simulink model "CDPRSim"  (R2023a)
settings: Solver=FixedStepAuto  StartTime=0.0  StopTime=inf  FixedStep=0.0001  RelTol=1e-3
values from neighbouring files (symbols this model uses):
  x11 = input('Enter x11 ')    [CDPRm.m]
  y11 = input('Enter y11 ')    [CDPRm.m]
undefined symbols (not defined in the file or in its folder): LBA, LTA, RBA, RTA
libraries: dspmathops x2, vrlib x1
(part 1 of 2)
settings Model: Creator=user  LastModifiedBy=omert
settings SolverCC: AlgebraicLoopSolver=TrustRegion
settings DataIOCC: ReturnWorkspaceOutputs=off
settings DebuggingCC: UnconnectedInputMsg=warning  UnconnectedOutputMsg=warning  UnconnectedLineMsg=warning  ArithmeticOperatorsInVariantConditions=warning
settings ModelReferenceCC: EnableRefExpFcnMdlSchedulingChecks=on
settings SFSimCC: CustomCodeUndefinedFunction=UseInterfaceOnly

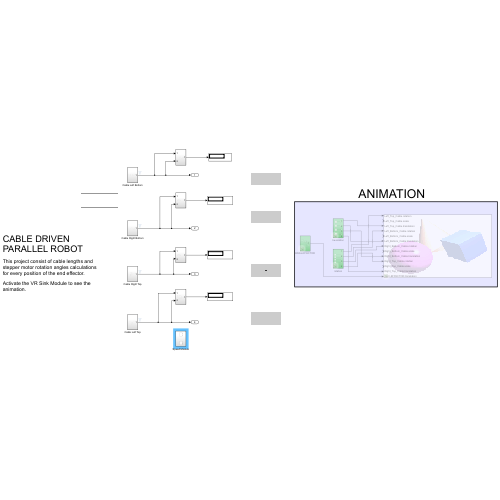
[thumbnail: Simulink's stored preview of the top-level diagram]
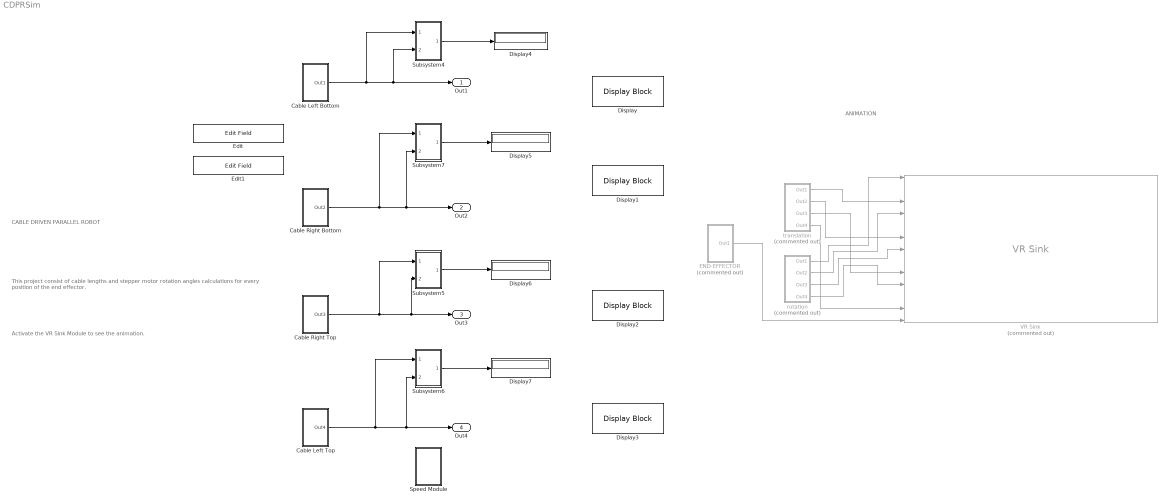
== system CDPRSim ==
  note: ANIMATION
  note: This project consist of cable lengths and stepper motor rotation angles calculations
      | for every position of the end effector.
  note: CABLE DRIVEN PARALLEL ROBOT
  note: Activate the VR Sink Module to see the
      | animation.
  Cable Left Bottom : Subsystem
  Cable Left Top : Subsystem
  Cable Right Bottom : Subsystem
  Cable Right Top : Subsystem
  Display{,1..3} (4 alike) : DisplayBlock  LabelPosition=Hide  Format=long
  Display{4..7} (4 alike) : Display
  END-EFFECTOR : Subsystem  Commented=on
  Edit : EditField  LabelPosition=Hide  ShowInitialText=on  Alignment=Center
  Edit1 : EditField  LabelPosition=Hide  ShowInitialText=on  Alignment=Center
  Speed Module : Subsystem
  Subsystem4 : Subsystem
  Subsystem5 : Subsystem
  Subsystem6 : Subsystem
  Subsystem7 : Subsystem
  VR Sink : vrlib/VR Sink  Commented=on  InstantiateOnLoad=on  SampleTime=0.00000000000000000000001  ViewEnable=on  RemoteChange=off  RemoteView=off  FieldsWritten=Left_Top_Cable.rotation.4.1.1.double#Left_Top_Cable.scale.3.1.1.double#Left_Top_Cable.translation.3.1.1.double#Left_Bottom_Cable.rotation.4.1.1.double#Left_Bottom_Cable.scale.3.1.1.double#Left_Bottom_Cable.translation.3.1.1.double#Right_Bottom_Cable.rotation.4.1.1.double#Right_Bottom_Cable.scale.3.1.1.double#Right_Bottom_Cable.translation.3.1.1.double#Right_Top_Cable.rotation.4.1.1.double#Right_Top_Cable.scale.3.1.1.double#Right_Top_Cable.translation.3.1.1.double#END-EFFECTOR.translation.3.1.1.double  WorldFileName=C:\Users\omert\OneDrive\Masaüstü\EFSANE.WRL  AutoView=off  VideoDimensions=[]  AllowVariableSize=off  FigureProperties="{'Position', 'Name', 'Viewpoint', 'CameraBound', 'CameraDirection', 'CameraPosition', 'CameraUpVector', 'ZoomFactor', 'Antialiasing', 'Headlight', 'Lighting', 'NavPanel', 'Sound', 'StatusBar', 'Stereo3D', 'Stereo3DCameraOffset', 'Stereo3DHIT', 'ToolBar', 'Textures', 'Transparency', 'Triad', 'Wireframe', 'NavZones', 'NavMode', 'NavSpeed', 'CaptureFileFormat', 'CaptureFileName', 'Record2DCompressMethod', 'Record2DCompressQuality', 'Record2D', 'Record2DFileName', 'Record2DFPS'; [9.8000000000000000e+02   8.4000000000000000e+01   3.8600000000000000e+02   5.9200000000000000e+02], '', '_untitled_1', 'on', [1.2435298260286720e-01  -4.3285041558913911e-02  -9.9129346860300416e-01], [-6.5430573152632743e+00   6.6945298656339713e-01   1.1992959271284654e+01], [-2.1811017115516454e-01   9.7342014038062419e-01  -6.9865467435618681e-02], [1.0000000000000000e+00], 'on', 'on', 'on', 'halfbar', 'on', 'on', 'off', [1.0000000149011612e-01], [0.0000000000000000e+00], 'on', 'on', 'on', 'none', 'on', 'off', 'examine', 'normal', 'tif', '%f_anim_%n.tif', 'auto', [7.5000000000000000e+01], 'off', '%f_anim_%n.avi', 'auto'}"
  rotation : Subsystem  Commented=on
  translation : Subsystem  Commented=on
  Out1 : Outport  VectorParamsAs1DForOutWhenUnconnected=off
  Out2 : Outport  Port=2  VectorParamsAs1DForOutWhenUnconnected=off
  Out3 : Outport  Port=3  VectorParamsAs1DForOutWhenUnconnected=off
  Out4 : Outport  Port=4  VectorParamsAs1DForOutWhenUnconnected=off
  wires:
  Cable Left Bottom/1(Out1) -> Out1/1, Subsystem4/2(In2), Subsystem4/1(In1)
  Cable Right Bottom/1(Out2) -> Subsystem7/1(In1), Out2/1, Subsystem7/2(In2)
  Cable Right Top/1(Out3) -> Subsystem5/1(In1), Subsystem5/2(In2), Out3/1
  Cable Left Top/1(Out4) -> Subsystem6/1(In1), Subsystem6/2(In2), Out4/1
  Subsystem4/1(Out1) -> Display4/1
  Subsystem5/1(Out1) -> Display6/1
  Subsystem6/1(Out1) -> Display7/1
  Subsystem7/1(Out1) -> Display5/1
  rotation/4(Out4) -> VR Sink/10
  rotation/1(Out1) -> VR Sink/1
  translation/3(Out3) -> VR Sink/9
  translation/1(Out1) -> VR Sink/3
  rotation/2(Out2) -> VR Sink/4
  translation/4(Out4) -> VR Sink/12
  translation/2(Out2) -> VR Sink/6
  rotation/3(Out3) -> VR Sink/7
  END-EFFECTOR/1(Out1) -> VR Sink/13

== system CDPRSim/Cable Left Bottom ==
  Constant1 : Constant
  Constant5 : Constant
  Gain : Gain  Gain=x11
  Gain1 : Gain  Gain=y11
  Sqrt2 : Sqrt
  Square : Math  Operator=square  SignedPower=on
  Square1 : Math  Operator=square  SignedPower=on
  Sum : Sum  Inputs=|++
  Out1 : Outport  VectorParamsAs1DForOutWhenUnconnected=off
  wires:
  Gain1/1 -> Square1/1
  Gain/1 -> Square/1
  Constant5/1 -> Gain1/1
  Square1/1 -> Sum/2
  Square/1 -> Sum/1
  Constant1/1 -> Gain/1
  Sum/1 -> Sqrt2/1
  Sqrt2/1 -> Out1/1

== system CDPRSim/Cable Left Top ==
  Constant{1..2,4..5} (4 alike) : Constant
  Gain : Gain  Gain=x11
  Gain1 : Gain  Gain=y11
  Gain4 : Gain  Gain=70
  Gain5 : Gain  Gain=1000
  Sqrt : Sqrt
  Square : Math  Operator=square  SignedPower=on
  Square1 : Math  Operator=square  SignedPower=on
  Sum : Sum  Inputs=|++
  Sum2 : Sum  Inputs=|+--
  Out4 : Outport  VectorParamsAs1DForOutWhenUnconnected=off
  wires:
  Square1/1 -> Sum/2
  Sum2/1 -> Square1/1
  Sum/1 -> Sqrt/1
  Gain5/1 -> Sum2/1
  Constant4/1 -> Gain4/1
  Gain1/1 -> Sum2/2
  Gain/1 -> Square/1
  Sqrt/1 -> Out4/1
  Constant1/1 -> Gain1/1
  Constant2/1 -> Gain/1
  Square/1 -> Sum/1
  Constant5/1 -> Gain5/1
  Gain4/1 -> Sum2/3

== system CDPRSim/Cable Right Bottom ==
  Constant{,1..3} (4 alike) : Constant
  Gain : Gain  Gain=x11
  Gain1 : Gain  Gain=y11
  Gain2 : Gain  Gain=1000
  Gain3 : Gain  Gain=70
  Sqrt : Sqrt
  Square : Math  Operator=square  SignedPower=on
  Square1 : Math  Operator=square  SignedPower=on
  Sum : Sum  Inputs=|++
  Sum1 : Sum  Inputs=|+--
  Out2 : Outport  VectorParamsAs1DForOutWhenUnconnected=off
  wires:
  Constant/1 -> Gain2/1
  Gain2/1 -> Sum1/1
  Square/1 -> Sum/1
  Constant1/1 -> Gain1/1
  Gain/1 -> Sum1/2
  Sum1/1 -> Square/1
  Square1/1 -> Sum/2
  Sqrt/1 -> Out2/1
  Gain1/1 -> Square1/1
  Sum/1 -> Sqrt/1
  Constant2/1 -> Gain/1
  Gain3/1 -> Sum1/3
  Constant3/1 -> Gain3/1

== system CDPRSim/Cable Right Top ==
  Constant{,1..5} (6 alike) : Constant
  Gain : Gain  Gain=x11
  Gain1 : Gain  Gain=y11
  Gain2 : Gain  Gain=1000
  Gain3 : Gain  Gain=70
  Gain4 : Gain  Gain=70
  Gain5 : Gain  Gain=1000
  Sqrt : Sqrt
  Square : Math  Operator=square  SignedPower=on
  Square1 : Math  Operator=square  SignedPower=on
  Sum : Sum  Inputs=|++
  Sum1 : Sum  Inputs=|+--
  Sum2 : Sum  Inputs=|+--
  Out3 : Outport  VectorParamsAs1DForOutWhenUnconnected=off
  wires:
  Constant4/1 -> Gain4/1
  Constant/1 -> Gain2/1
  Gain/1 -> Sum1/2
  Sqrt/1 -> Out3/1
  Constant3/1 -> Gain3/1
  Constant2/1 -> Gain/1
  Sum1/1 -> Square/1
  Square/1 -> Sum/1
  Gain1/1 -> Sum2/2
  Square1/1 -> Sum/2
  Gain2/1 -> Sum1/1
  Gain3/1 -> Sum1/3
  Sum/1 -> Sqrt/1
  Constant1/1 -> Gain1/1
  Gain4/1 -> Sum2/3
  Constant5/1 -> Gain5/1
  Gain5/1 -> Sum2/1
  Sum2/1 -> Square1/1

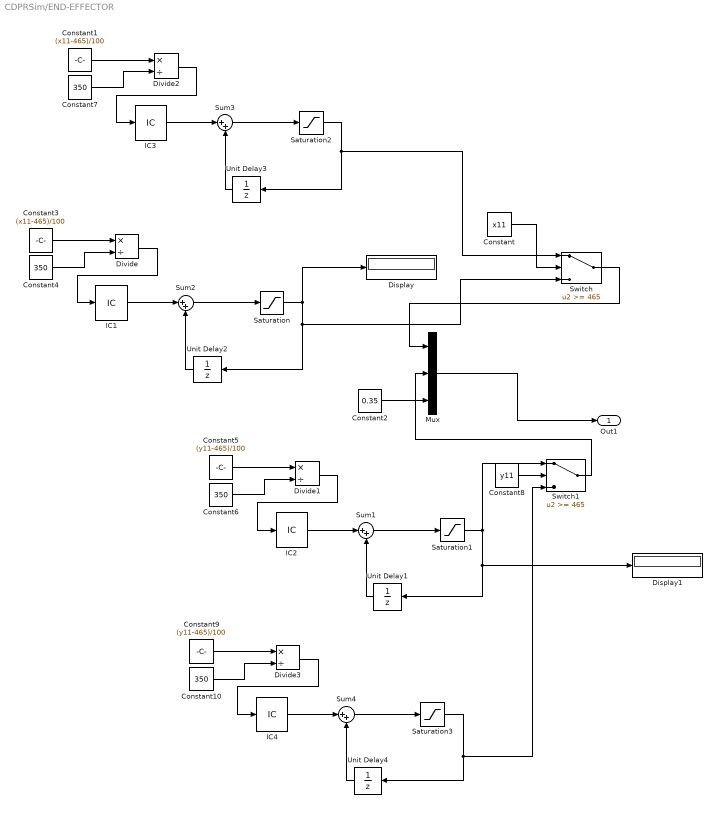
== system CDPRSim/END-EFFECTOR ==
  Constant : Constant  Value=x11
  Constant1 : Constant  Value=(x11-465)/100
  Constant{4,6..7,10} (4 alike) : Constant  Value=350
  Constant2 : Constant  Value=0.35
  Constant3 : Constant  Value=(x11-465)/100
  Constant5 : Constant  Value=(y11-465)/100
  Constant8 : Constant  Value=y11
  Constant9 : Constant  Value=(y11-465)/100
  Display : Display
  Display1 : Display
  Divide{,1..3} (4 alike) : Product  Inputs=*/
  IC{1..4} (4 alike) : InitialCondition  Value=0
  Mux : Mux  Inputs=3
  Saturation : Saturate  UpperLimit=inf  LowerLimit=(x11-465)/100
  Saturation1 : Saturate  UpperLimit=(y11-465)/100  LowerLimit=-inf
  Saturation2 : Saturate  UpperLimit=(x11-465)/100  LowerLimit=-inf
  Saturation3 : Saturate  UpperLimit=inf  LowerLimit=(y11-465)/100
  Sum{1..4} (4 alike) : Sum  Inputs=|++
  Switch : Switch  Threshold=465  SaturateOnIntegerOverflow=off  InputSameDT=off
  Switch1 : Switch  Threshold=465  SaturateOnIntegerOverflow=off  InputSameDT=off
  Unit Delay{1..4} (4 alike) : UnitDelay  SampleTime=-1  HasFrameUpgradeWarning=on
  Out1 : Outport
  wires:
  Saturation/1 -> Unit Delay2/1, Switch/3, Display/1
  Mux/1 -> Out1/1
  Constant2/1 -> Mux/3
  IC1/1 -> Sum2/1
  Unit Delay2/1 -> Sum2/2
  Sum2/1 -> Saturation/1
  Constant3/1 -> Divide/1
  Constant4/1 -> Divide/2
  Divide/1 -> IC1/1
  Divide1/1 -> IC2/1
  Sum1/1 -> Saturation1/1
  Constant6/1 -> Divide1/2
  Unit Delay1/1 -> Sum1/2
  Constant5/1 -> Divide1/1
  IC2/1 -> Sum1/1
  Saturation1/1 -> Display1/1, Unit Delay1/1, Switch1/1
  Constant/1 -> Switch/2
  Switch/1 -> Mux/1
  Sum3/1 -> Saturation2/1
  Unit Delay3/1 -> Sum3/2
  Divide2/1 -> IC3/1
  Constant7/1 -> Divide2/2
  Saturation2/1 -> Switch/1, Unit Delay3/1
  Constant1/1 -> Divide2/1
  IC3/1 -> Sum3/1
  Switch1/1 -> Mux/2
  Constant8/1 -> Switch1/2
  Constant9/1 -> Divide3/1
  IC4/1 -> Sum4/1
  Unit Delay4/1 -> Sum4/2
  Sum4/1 -> Saturation3/1
  Constant10/1 -> Divide3/2
  Divide3/1 -> IC4/1
  Saturation3/1 -> Switch1/3, Unit Delay4/1

== system CDPRSim/Speed Module ==
  "Left bottom hız " : Subsystem
  Subsystem : Subsystem

== system CDPRSim/Subsystem4 ==
  In1 : Inport
  In2 : Inport  Port=2
  Display : Display
  Relational Operator : RelationalOperator  Operator===  OutDataTypeStr=boolean  RndMeth=Simplest  InputSameDT=off
  Sum2 : Sum  Inputs=|+-
  Triggered Subsystem : Subsystem  TreatAsAtomicUnit=on
  Unit Delay : UnitDelay  SampleTime=-1  HasFrameUpgradeWarning=on
  Out1 : Outport  VectorParamsAs1DForOutWhenUnconnected=off
  wires:
  In1/1 -> Sum2/1, Unit Delay/1
  Unit Delay/1 -> Triggered Subsystem/1(In1), Relational Operator/2
  Sum2/1 -> Display/1, Out1/1
  Triggered Subsystem/1(Out1) -> Sum2/2
  Relational Operator/1 -> Triggered Subsystem/Trigger
  In2/1 -> Relational Operator/1

== system CDPRSim/Subsystem5 ==
  In1 : Inport
  In2 : Inport  Port=2
  Relational Operator2 : RelationalOperator  Operator===  OutDataTypeStr=boolean  RndMeth=Simplest  InputSameDT=off
  Sum3 : Sum  Inputs=|+-
  Triggered Subsystem2 : Subsystem  TreatAsAtomicUnit=on
  Unit Delay2 : UnitDelay  SampleTime=-1  HasFrameUpgradeWarning=on
  Out1 : Outport  VectorParamsAs1DForOutWhenUnconnected=off
  wires:
  Unit Delay2/1 -> Triggered Subsystem2/1(In1), Relational Operator2/2
  Sum3/1 -> Out1/1
  Relational Operator2/1 -> Triggered Subsystem2/Trigger
  In1/1 -> Unit Delay2/1, Sum3/1
  Triggered Subsystem2/1(Out1) -> Sum3/2
  In2/1 -> Relational Operator2/1

== system CDPRSim/Subsystem6 ==
  In1 : Inport
  In2 : Inport  Port=2
  Relational Operator3 : RelationalOperator  Operator===  OutDataTypeStr=boolean  RndMeth=Simplest  InputSameDT=off
  Sum4 : Sum  Inputs=|+-
  Triggered Subsystem3 : Subsystem  TreatAsAtomicUnit=on
  Unit Delay3 : UnitDelay  SampleTime=-1  HasFrameUpgradeWarning=on
  Out1 : Outport  VectorParamsAs1DForOutWhenUnconnected=off
  wires:
  In1/1 -> Unit Delay3/1, Sum4/1
  Unit Delay3/1 -> Relational Operator3/2, Triggered Subsystem3/1(In1)
  Sum4/1 -> Out1/1
  Triggered Subsystem3/1(Out1) -> Sum4/2
  Relational Operator3/1 -> Triggered Subsystem3/Trigger
  In2/1 -> Relational Operator3/1

== system CDPRSim/Subsystem7 ==
  In1 : Inport
  In2 : Inport  Port=2
  Relational Operator1 : RelationalOperator  Operator===  OutDataTypeStr=boolean  RndMeth=Simplest  InputSameDT=off
  Sum1 : Sum  Inputs=|+-
  Triggered Subsystem1 : Subsystem  TreatAsAtomicUnit=on
  Unit Delay1 : UnitDelay  SampleTime=-1  HasFrameUpgradeWarning=on
  Out1 : Outport  VectorParamsAs1DForOutWhenUnconnected=off
  wires:
  In1/1 -> Sum1/1, Unit Delay1/1
  Sum1/1 -> Out1/1
  Unit Delay1/1 -> Relational Operator1/2, Triggered Subsystem1/1(In1)
  In2/1 -> Relational Operator1/1
  Relational Operator1/1 -> Triggered Subsystem1/Trigger
  Triggered Subsystem1/1(Out1) -> Sum1/2

== system CDPRSim/rotation ==
  LEFT TOP : Subsystem
  LEFT-BOTTOM : Subsystem
  RIGHT-BOTTOM : Subsystem
  RIGHT-TOP : Subsystem
  Out1 : Outport
  Out2 : Outport  Port=2
  Out3 : Outport  Port=3
  Out4 : Outport  Port=4
  wires:
  RIGHT-TOP/1(Out1) -> Out4/1
  LEFT-BOTTOM/1(Out1) -> Out2/1
  RIGHT-BOTTOM/1(Out1) -> Out3/1
  LEFT TOP/1(Out1) -> Out1/1

== system CDPRSim/translation ==
  LEFT BOTTOM : Subsystem
  LEFT TOP : Subsystem
  RIGHT TOP : Subsystem
  RIGHT-BOTTOM : Subsystem
  Out1 : Outport
  Out2 : Outport  Port=2
  Out3 : Outport  Port=3
  Out4 : Outport  Port=4
  wires:
  RIGHT TOP/1(Out1) -> Out4/1
  LEFT TOP/1(Out1) -> Out1/1
  RIGHT-BOTTOM/1(Out1) -> Out3/1
  LEFT BOTTOM/1(Out1) -> Out2/1

== system CDPRSim/Speed Module/Left bottom hız  ==
  Abs : Abs  SaturateOnIntegerOverflow=off
  Cumulative Sum : dspmathops/Cumulative Sum  dim=Channels (running sum)  InputProcessing=Columns as channels (frame based)  reset_popup=None  roundingMode=Floor  overflowMode=off  outputDataTypeStr=Inherit: Same as accumulator  outputMin=[]  outputMax=[]  outputLastDataTypeStr=Inherit: Same as accumulator
  Display{1..4,6} (5 alike) : Display
  "Fark " : Subsystem
  Sum : Sum  Inputs=|+-
  Unit Delay : UnitDelay  SampleTime=-1  HasFrameUpgradeWarning=on
  constant : Subsystem
  "slope " : Subsystem
  x2-x1 : Subsystem
  y value : Subsystem
  y2-y1 : Subsystem
  "yeni uzunluklar " : Subsystem
  Out1 : Outport  VectorParamsAs1DForOutWhenUnconnected=off
  Out2 : Outport  Port=2  VectorParamsAs1DForOutWhenUnconnected=off
  wires:
  constant/1(Out1) -> y value/2("constant ")
  "Fark "/1(Out1) -> Display1/1
  "slope "/1(Out1) -> Display3/1, y value/1("slope "), constant/1(In1)
  Cumulative Sum/1 -> "Fark "/1(In1), Display6/1
  Unit Delay/1 -> Sum/2
  Sum/1 -> Display4/1, Abs/1
  x2-x1/2(Out1) -> "slope "/2(In2)
  y2-y1/2(Out2) -> "slope "/1(In1)
  Abs/1 -> Cumulative Sum/1
  y2-y1/1(Out1) -> Out1/1
  x2-x1/1(Out6) -> Out2/1
  "yeni uzunluklar "/1(Out1) -> Unit Delay/1, Sum/1, Display2/1
  y value/1(Out1) -> "yeni uzunluklar "/1(In1)

== system CDPRSim/Speed Module/Subsystem ==
  Abs : Abs  SaturateOnIntegerOverflow=off
  Cumulative Sum : dspmathops/Cumulative Sum  dim=Channels (running sum)  InputProcessing=Columns as channels (frame based)  reset_popup=None  roundingMode=Floor  overflowMode=off  outputDataTypeStr=Inherit: Same as accumulator  outputMin=[]  outputMax=[]  outputLastDataTypeStr=Inherit: Same as accumulator
  Display{1..5} (5 alike) : Display
  "Fark " : Subsystem
  Sum : Sum  Inputs=|+-
  Unit Delay : UnitDelay  SampleTime=-1  HasFrameUpgradeWarning=on
  constant : Subsystem
  "slope " : Subsystem
  x2-x1 : Subsystem
  y value : Subsystem
  y2-y1 : Subsystem
  "yeni uzunluklar " : Subsystem
  Out1 : Outport  VectorParamsAs1DForOutWhenUnconnected=off
  Out2 : Outport  Port=2  VectorParamsAs1DForOutWhenUnconnected=off
  wires:
  Sum/1 -> Display4/1, Abs/1
  x2-x1/2(Out1) -> "slope "/2(In2)
  x2-x1/1(Out6) -> Out2/1
  y2-y1/1(Out1) -> Out1/1
  "yeni uzunluklar "/1(Out1) -> Unit Delay/1, Sum/1, Display2/1
  "slope "/1(Out1) -> Display3/1, constant/1(In1), y value/1("slope ")
  Unit Delay/1 -> Sum/2
  y value/1(Out1) -> "yeni uzunluklar "/1(In1), Display5/1
  "Fark "/1(Out1) -> Display1/1
  Cumulative Sum/1 -> "Fark "/1(In1)
  y2-y1/2(Out2) -> "slope "/1(In1)
  constant/1(Out1) -> y value/2("constant ")
  Abs/1 -> Cumulative Sum/1

== system CDPRSim/Subsystem4/Triggered Subsystem ==
  In1 : Inport
  Trigger : TriggerPort  TriggerType=falling  VariantControl=Variant
  Out1 : Outport  VectorParamsAs1DForOutWhenUnconnected=off
  wires:
  In1/1 -> Out1/1

== system CDPRSim/Subsystem5/Triggered Subsystem2 ==
  In1 : Inport
  Trigger : TriggerPort  TriggerType=falling  VariantControl=Variant
  Out1 : Outport  VectorParamsAs1DForOutWhenUnconnected=off
  wires:
  In1/1 -> Out1/1

== system CDPRSim/Subsystem6/Triggered Subsystem3 ==
  In1 : Inport
  Trigger : TriggerPort  TriggerType=falling  VariantControl=Variant
  Out1 : Outport  VectorParamsAs1DForOutWhenUnconnected=off
  wires:
  In1/1 -> Out1/1

== system CDPRSim/Subsystem7/Triggered Subsystem1 ==
  In1 : Inport
  Trigger : TriggerPort  TriggerType=falling  VariantControl=Variant
  Out1 : Outport  VectorParamsAs1DForOutWhenUnconnected=off
  wires:
  In1/1 -> Out1/1

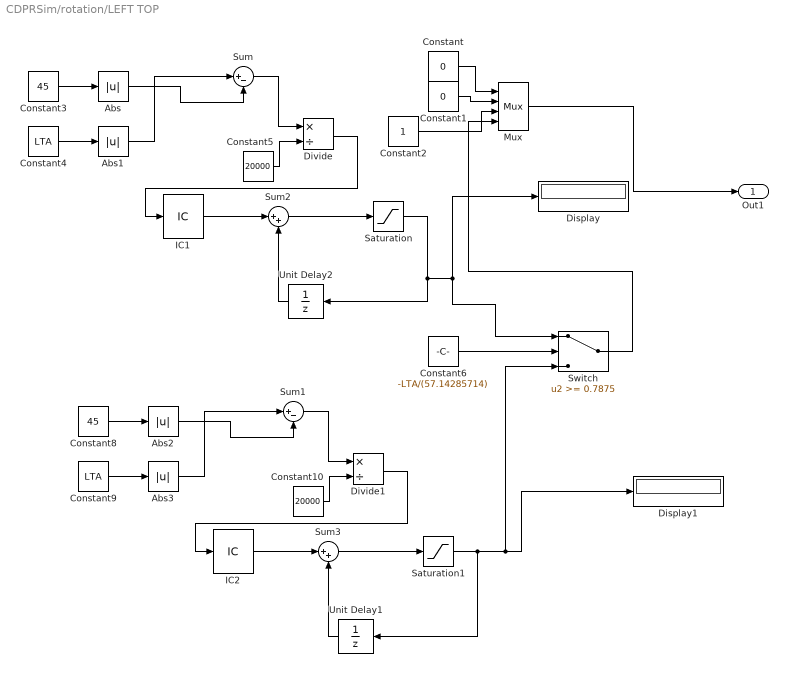
== system CDPRSim/rotation/LEFT TOP ==
  Abs{,1..3} (4 alike) : Abs  SaturateOnIntegerOverflow=off
  Constant : Constant  Value=0
  Constant1 : Constant  Value=0
  Constant10 : Constant  Value=20000
  Constant2 : Constant
  Constant3 : Constant  Value=45
  Constant4 : Constant  Value=LTA
  Constant5 : Constant  Value=20000
  Constant6 : Constant  Value=-LTA/(57.14285714)
  Constant8 : Constant  Value=45
  Constant9 : Constant  Value=LTA
  Display : Display
  Display1 : Display
  Divide : Product  Inputs=*/
  Divide1 : Product  Inputs=*/
  IC1 : InitialCondition  Value=0.7875
  IC2 : InitialCondition  Value=0.7875
  Mux : Mux
  Saturation : Saturate  UpperLimit=-LTA/(57.14285714)  LowerLimit=-inf
  Saturation1 : Saturate  UpperLimit=inf  LowerLimit=-LTA/(57.14285714)
  Sum : Sum  Inputs=|+-
  Sum1 : Sum  Inputs=|+-
  Sum2 : Sum  Inputs=|++
  Sum3 : Sum  Inputs=|++
  Switch : Switch  Threshold=0.7875  SaturateOnIntegerOverflow=off  InputSameDT=off
  Unit Delay1 : UnitDelay  SampleTime=-1  HasFrameUpgradeWarning=on
  Unit Delay2 : UnitDelay  SampleTime=-1  HasFrameUpgradeWarning=on
  Out1 : Outport
  wires:
  Mux/1 -> Out1/1
  Constant/1 -> Mux/1
  Constant1/1 -> Mux/2
  Constant2/1 -> Mux/3
  Unit Delay2/1 -> Sum2/2
  Sum2/1 -> Saturation/1
  IC1/1 -> Sum2/1
  Saturation/1 -> Display/1, Switch/1, Unit Delay2/1
  Constant4/1 -> Abs1/1
  Constant3/1 -> Abs/1
  Sum/1 -> Divide/1
  Constant5/1 -> Divide/2
  Divide/1 -> IC1/1
  Abs/1 -> Sum/2
  Abs1/1 -> Sum/1
  Constant6/1 -> Switch/2
  Switch/1 -> Mux/4
  IC2/1 -> Sum3/1
  Unit Delay1/1 -> Sum3/2
  Constant10/1 -> Divide1/2
  Constant9/1 -> Abs3/1
  Sum1/1 -> Divide1/1
  Constant8/1 -> Abs2/1
  Abs3/1 -> Sum1/1
  Sum3/1 -> Saturation1/1
  Abs2/1 -> Sum1/2
  Divide1/1 -> IC2/1
  Saturation1/1 -> Switch/3, Display1/1, Unit Delay1/1

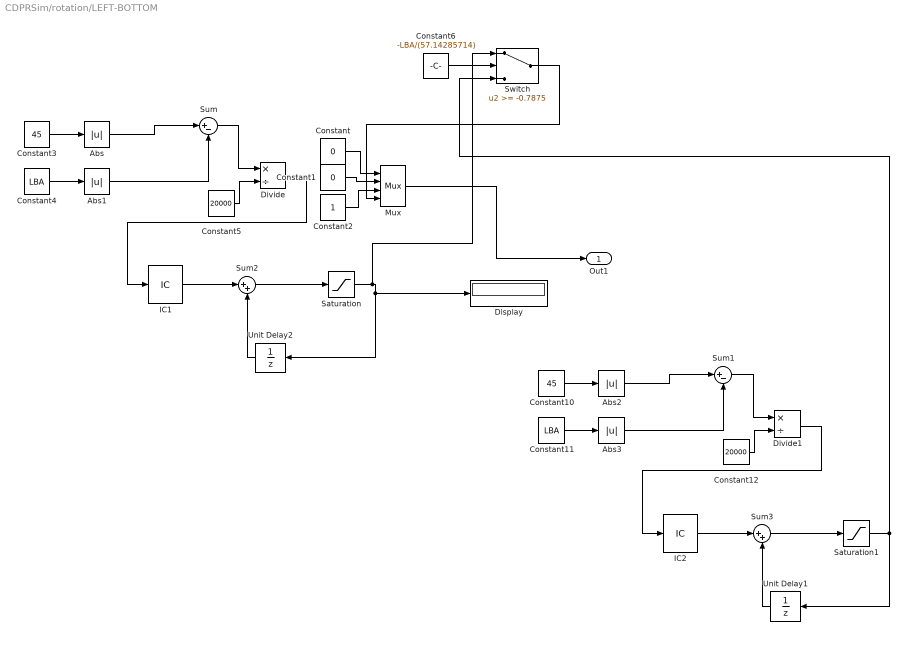
== system CDPRSim/rotation/LEFT-BOTTOM ==
  Abs{,1..3} (4 alike) : Abs  SaturateOnIntegerOverflow=off
  Constant : Constant  Value=0
  Constant1 : Constant  Value=0
  Constant10 : Constant  Value=45
  Constant11 : Constant  Value=LBA
  Constant12 : Constant  Value=20000
  Constant2 : Constant
  Constant3 : Constant  Value=45
  Constant4 : Constant  Value=LBA
  Constant5 : Constant  Value=20000
  Constant6 : Constant  Value=-LBA/(57.14285714)
  Display : Display
  Divide : Product  Inputs=*/
  Divide1 : Product  Inputs=*/
  IC1 : InitialCondition  Value=-0.7875
  IC2 : InitialCondition  Value=-0.7875
  Mux : Mux
  Saturation : Saturate  UpperLimit=-LBA/(57.14285714)  LowerLimit=-inf
  Saturation1 : Saturate  UpperLimit=inf  LowerLimit=-LBA/(57.14285714)
  Sum : Sum  Inputs=|+-
  Sum1 : Sum  Inputs=|+-
  Sum2 : Sum  Inputs=|++
  Sum3 : Sum  Inputs=|++
  Switch : Switch  Threshold=-0.7875  SaturateOnIntegerOverflow=off  InputSameDT=off
  Unit Delay1 : UnitDelay  SampleTime=-1  HasFrameUpgradeWarning=on
  Unit Delay2 : UnitDelay  SampleTime=-1  HasFrameUpgradeWarning=on
  Out1 : Outport
  wires:
  Constant2/1 -> Mux/3
  Constant1/1 -> Mux/2
  Constant/1 -> Mux/1
  Mux/1 -> Out1/1
  Unit Delay2/1 -> Sum2/2
  Sum2/1 -> Saturation/1
  IC1/1 -> Sum2/1
  Saturation/1 -> Switch/1, Display/1, Unit Delay2/1
  Constant5/1 -> Divide/2
  Constant4/1 -> Abs1/1
  Sum/1 -> Divide/1
  Constant3/1 -> Abs/1
  Divide/1 -> IC1/1
  Abs/1 -> Sum/1
  Abs1/1 -> Sum/2
  Constant6/1 -> Switch/2
  Switch/1 -> Mux/4
  Saturation1/1 -> Unit Delay1/1, Switch/3
  Divide1/1 -> IC2/1
  Sum1/1 -> Divide1/1
  Constant12/1 -> Divide1/2
  IC2/1 -> Sum3/1
  Sum3/1 -> Saturation1/1
  Unit Delay1/1 -> Sum3/2
  Abs3/1 -> Sum1/2
  Abs2/1 -> Sum1/1
  Constant11/1 -> Abs3/1
  Constant10/1 -> Abs2/1

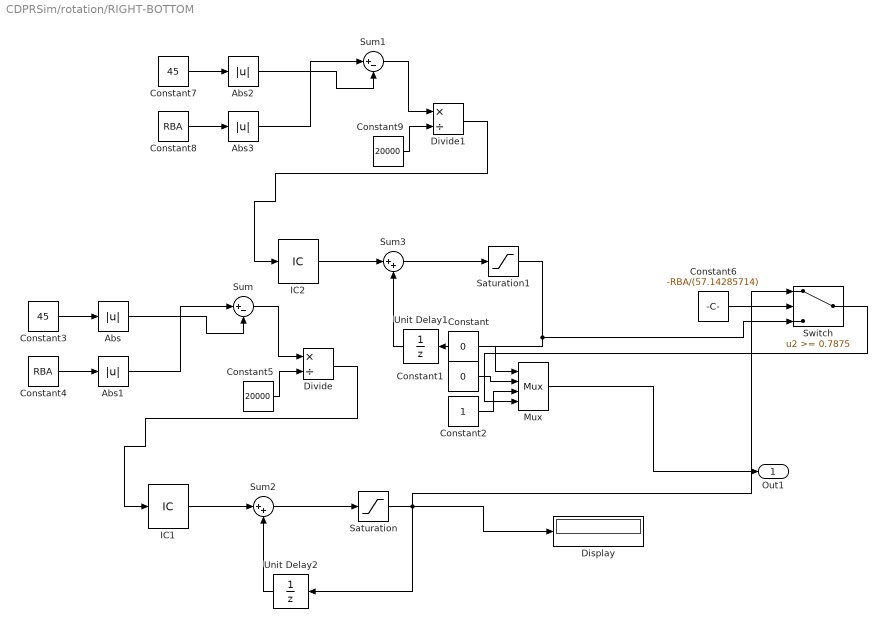
== system CDPRSim/rotation/RIGHT-BOTTOM ==
  Abs{,1..3} (4 alike) : Abs  SaturateOnIntegerOverflow=off
  Constant : Constant  Value=0
  Constant1 : Constant  Value=0
  Constant2 : Constant
  Constant3 : Constant  Value=45
  Constant4 : Constant  Value=RBA
  Constant5 : Constant  Value=20000
  Constant6 : Constant  Value=-RBA/(57.14285714)
  Constant7 : Constant  Value=45
  Constant8 : Constant  Value=RBA
  Constant9 : Constant  Value=20000
  Display : Display
  Divide : Product  Inputs=*/
  Divide1 : Product  Inputs=*/
  IC1 : InitialCondition  Value=0.7875
  IC2 : InitialCondition  Value=0.7875
  Mux : Mux
  Saturation : Saturate  UpperLimit=-RBA/(57.14285714)  LowerLimit=-inf
  Saturation1 : Saturate  UpperLimit=inf  LowerLimit=-RBA/(57.14285714)
  Sum : Sum  Inputs=|+-
  Sum1 : Sum  Inputs=|+-
  Sum2 : Sum  Inputs=|++
  Sum3 : Sum  Inputs=|++
  Switch : Switch  Threshold=0.7875  SaturateOnIntegerOverflow=off  InputSameDT=off
  Unit Delay1 : UnitDelay  SampleTime=-1  HasFrameUpgradeWarning=on
  Unit Delay2 : UnitDelay  SampleTime=-1  HasFrameUpgradeWarning=on
  Out1 : Outport
  wires:
  Constant2/1 -> Mux/3
  Constant1/1 -> Mux/2
  Constant/1 -> Mux/1
  Mux/1 -> Out1/1
  Unit Delay2/1 -> Sum2/2
  Sum2/1 -> Saturation/1
  IC1/1 -> Sum2/1
  Saturation/1 -> Switch/1, Display/1, Unit Delay2/1
  Constant5/1 -> Divide/2
  Constant4/1 -> Abs1/1
  Sum/1 -> Divide/1
  Constant3/1 -> Abs/1
  Divide/1 -> IC1/1
  Abs1/1 -> Sum/1
  Abs/1 -> Sum/2
  Constant6/1 -> Switch/2
  Switch/1 -> Mux/4
  IC2/1 -> Sum3/1
  Sum3/1 -> Saturation1/1
  Unit Delay1/1 -> Sum3/2
  Constant9/1 -> Divide1/2
  Sum1/1 -> Divide1/1
  Divide1/1 -> IC2/1
  Constant7/1 -> Abs2/1
  Constant8/1 -> Abs3/1
  Abs3/1 -> Sum1/1
  Saturation1/1 -> Switch/3, Unit Delay1/1
  Abs2/1 -> Sum1/2

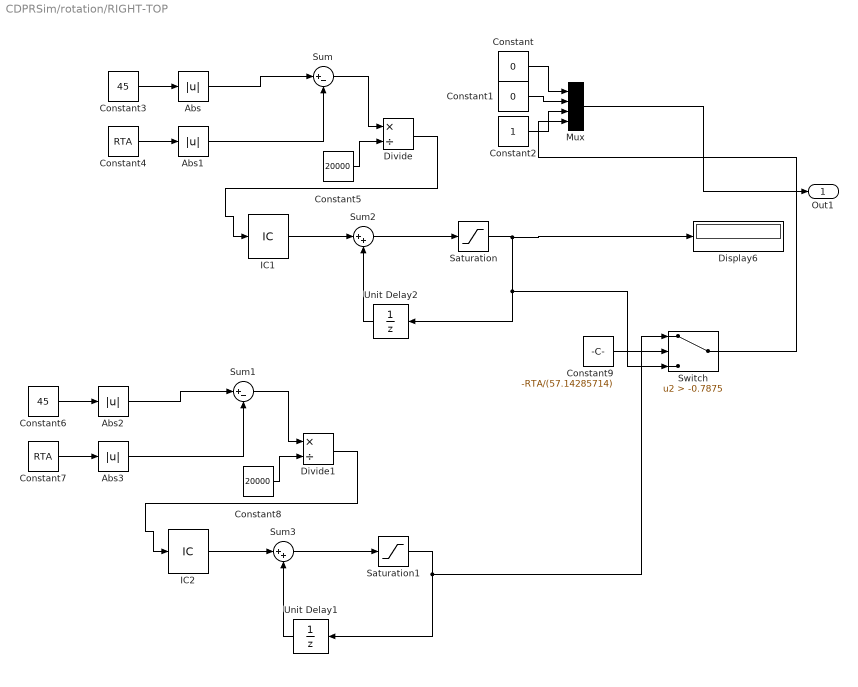
== system CDPRSim/rotation/RIGHT-TOP ==
  Abs{,1..3} (4 alike) : Abs  SaturateOnIntegerOverflow=off
  Constant : Constant  Value=0
  Constant1 : Constant  Value=0
  Constant2 : Constant
  Constant3 : Constant  Value=45
  Constant4 : Constant  Value=RTA
  Constant5 : Constant  Value=20000
  Constant6 : Constant  Value=45
  Constant7 : Constant  Value=RTA
  Constant8 : Constant  Value=20000
  Constant9 : Constant  Value=-RTA/(57.14285714)
  Display6 : Display
  Divide : Product  Inputs=*/
  Divide1 : Product  Inputs=*/
  IC1 : InitialCondition  Value=-0.7875
  IC2 : InitialCondition  Value=-0.7875
  Mux : Mux
  Saturation : Saturate  UpperLimit=inf  LowerLimit=-RTA/(57.14285714)
  Saturation1 : Saturate  UpperLimit=-RTA/(57.14285714)  LowerLimit=-inf
  Sum : Sum  Inputs=|+-
  Sum1 : Sum  Inputs=|+-
  Sum2 : Sum  Inputs=|++
  Sum3 : Sum  Inputs=|++
  Switch : Switch  Criteria=u2 > Threshold  Threshold=-0.7875  SaturateOnIntegerOverflow=off  InputSameDT=off
  Unit Delay1 : UnitDelay  SampleTime=-1  HasFrameUpgradeWarning=on
  Unit Delay2 : UnitDelay  SampleTime=-1  HasFrameUpgradeWarning=on
  Out1 : Outport
  wires:
  Constant2/1 -> Mux/3
  Constant1/1 -> Mux/2
  Constant/1 -> Mux/1
  Mux/1 -> Out1/1
  IC1/1 -> Sum2/1
  Unit Delay2/1 -> Sum2/2
  Sum2/1 -> Saturation/1
  Saturation/1 -> Display6/1, Switch/3, Unit Delay2/1
  Constant5/1 -> Divide/2
  Constant4/1 -> Abs1/1
  Sum/1 -> Divide/1
  Abs1/1 -> Sum/2
  Constant3/1 -> Abs/1
  Divide/1 -> IC1/1
  Abs/1 -> Sum/1
  Switch/1 -> Mux/4
  IC2/1 -> Sum3/1
  Saturation1/1 -> Switch/1, Unit Delay1/1
  Abs2/1 -> Sum1/1
  Sum1/1 -> Divide1/1
  Constant7/1 -> Abs3/1
  Constant8/1 -> Divide1/2
  Unit Delay1/1 -> Sum3/2
  Divide1/1 -> IC2/1
  Sum3/1 -> Saturation1/1
  Constant6/1 -> Abs2/1
  Abs3/1 -> Sum1/2
  Constant9/1 -> Switch/2

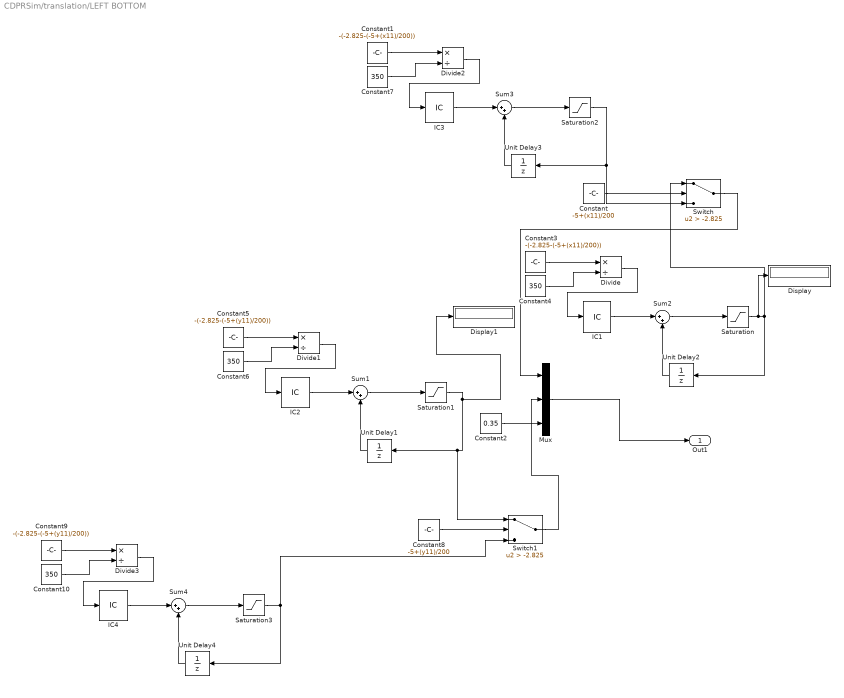
== system CDPRSim/translation/LEFT BOTTOM ==
  Constant : Constant  Value=-5+(x11)/200
  Constant1 : Constant  Value=-(-2.825-(-5+(x11)/200))
  Constant{4,6..7,10} (4 alike) : Constant  Value=350
  Constant2 : Constant  Value=0.35
  Constant3 : Constant  Value=-(-2.825-(-5+(x11)/200))
  Constant5 : Constant  Value=-(-2.825-(-5+(y11)/200))
  Constant8 : Constant  Value=-5+(y11)/200
  Constant9 : Constant  Value=-(-2.825-(-5+(y11)/200))
  Display : Display
  Display1 : Display
  Divide{,1..3} (4 alike) : Product  Inputs=*/
  IC{1..4} (4 alike) : InitialCondition  Value=-2.825
  Mux : Mux  Inputs=3
  Saturation : Saturate  UpperLimit=-5+(x11)/200  LowerLimit=-inf
  Saturation1 : Saturate  UpperLimit=-5+(y11)/200  LowerLimit=-inf
  Saturation2 : Saturate  UpperLimit=inf  LowerLimit=-5+(x11)/200
  Saturation3 : Saturate  UpperLimit=inf  LowerLimit=-5+(y11)/200
  Sum{1..4} (4 alike) : Sum  Inputs=|++
  Switch : Switch  Criteria=u2 > Threshold  Threshold=-2.825  SaturateOnIntegerOverflow=off  InputSameDT=off
  Switch1 : Switch  Criteria=u2 > Threshold  Threshold=-2.825  SaturateOnIntegerOverflow=off  InputSameDT=off
  Unit Delay{1..4} (4 alike) : UnitDelay  SampleTime=-1  HasFrameUpgradeWarning=on
  Out1 : Outport
  wires:
  Mux/1 -> Out1/1
  Constant2/1 -> Mux/3
  Saturation1/1 -> Switch1/1, Unit Delay1/1, Display1/1
  Unit Delay2/1 -> Sum2/2
  Sum2/1 -> Saturation/1
  IC1/1 -> Sum2/1
  Saturation/1 -> Display/1, Unit Delay2/1, Switch/1
  Constant3/1 -> Divide/1
  Divide/1 -> IC1/1
  Constant4/1 -> Divide/2
  Unit Delay1/1 -> Sum1/2
  IC2/1 -> Sum1/1
  Constant5/1 -> Divide1/1
  Constant6/1 -> Divide1/2
  Divide1/1 -> IC2/1
  Sum1/1 -> Saturation1/1
  Constant/1 -> Switch/2
  Switch/1 -> Mux/1
  Saturation2/1 -> Switch/3, Unit Delay3/1
  Divide2/1 -> IC3/1
  Constant1/1 -> Divide2/1
  IC3/1 -> Sum3/1
  Constant7/1 -> Divide2/2
  Sum3/1 -> Saturation2/1
  Unit Delay3/1 -> Sum3/2
  Constant8/1 -> Switch1/2
  Switch1/1 -> Mux/2
  Constant10/1 -> Divide3/2
  Unit Delay4/1 -> Sum4/2
  Divide3/1 -> IC4/1
  Sum4/1 -> Saturation3/1
  Constant9/1 -> Divide3/1
  Saturation3/1 -> Unit Delay4/1, Switch1/3
  IC4/1 -> Sum4/1

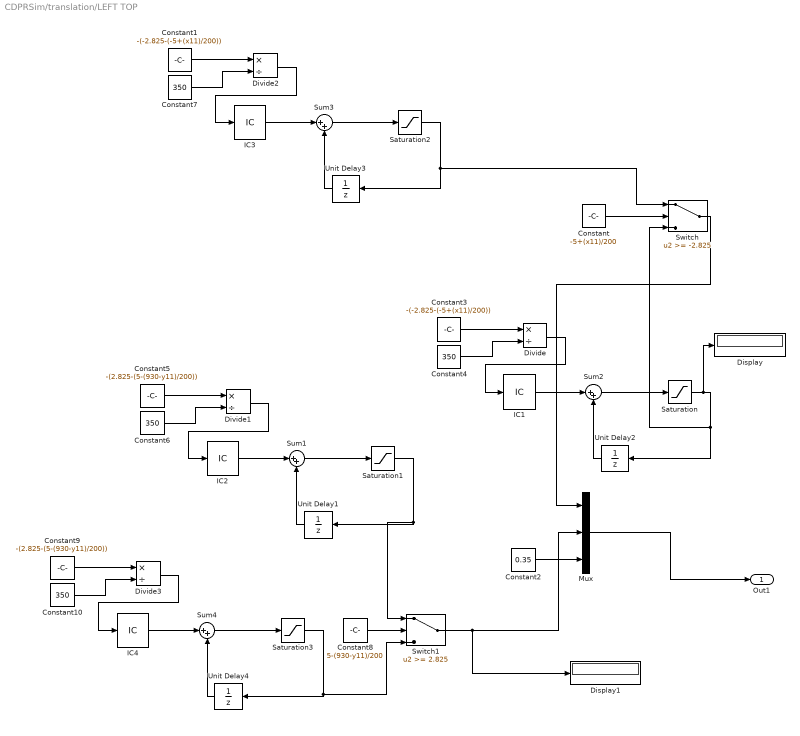
== system CDPRSim/translation/LEFT TOP ==
  Constant : Constant  Value=-5+(x11)/200
  Constant1 : Constant  Value=-(-2.825-(-5+(x11)/200))
  Constant{4,6..7,10} (4 alike) : Constant  Value=350
  Constant2 : Constant  Value=0.35
  Constant3 : Constant  Value=-(-2.825-(-5+(x11)/200))
  Constant5 : Constant  Value=-(2.825-(5-(930-y11)/200))
  Constant8 : Constant  Value=5-(930-y11)/200
  Constant9 : Constant  Value=-(2.825-(5-(930-y11)/200))
  Display : Display
  Display1 : Display
  Divide{,1..3} (4 alike) : Product  Inputs=*/
  IC1 : InitialCondition  Value=-2.825
  IC2 : InitialCondition  Value=2.825
  IC3 : InitialCondition  Value=-2.825
  IC4 : InitialCondition  Value=2.825
  Mux : Mux  Inputs=3
  Saturation : Saturate  UpperLimit=inf  LowerLimit=-5+(x11)/200
  Saturation1 : Saturate  UpperLimit=5-(930-y11)/200  LowerLimit=-inf
  Saturation2 : Saturate  UpperLimit=-5+(x11)/200  LowerLimit=-inf
  Saturation3 : Saturate  UpperLimit=inf  LowerLimit=5-(930-y11)/200
  Sum{1..4} (4 alike) : Sum  Inputs=|++
  Switch : Switch  Threshold=-2.825  SaturateOnIntegerOverflow=off  InputSameDT=off
  Switch1 : Switch  Threshold=2.825  SaturateOnIntegerOverflow=off  InputSameDT=off
  Unit Delay{1..4} (4 alike) : UnitDelay  SampleTime=-1  HasFrameUpgradeWarning=on
  Out1 : Outport
  wires:
  Constant2/1 -> Mux/3
  Mux/1 -> Out1/1
  Divide/1 -> IC1/1
  Sum2/1 -> Saturation/1
  Constant4/1 -> Divide/2
  Unit Delay2/1 -> Sum2/2
  Saturation/1 -> Display/1, Switch/3, Unit Delay2/1
  IC1/1 -> Sum2/1
  Constant3/1 -> Divide/1
  Unit Delay1/1 -> Sum1/2
  Sum1/1 -> Saturation1/1
  IC2/1 -> Sum1/1
  Saturation1/1 -> Switch1/1, Unit Delay1/1
  Constant5/1 -> Divide1/1
  Divide1/1 -> IC2/1
  Constant6/1 -> Divide1/2
  Constant/1 -> Switch/2
  Switch/1 -> Mux/1
  Unit Delay3/1 -> Sum3/2
  Sum3/1 -> Saturation2/1
  IC3/1 -> Sum3/1
  Saturation2/1 -> Switch/1, Unit Delay3/1
  Constant1/1 -> Divide2/1
  Divide2/1 -> IC3/1
  Constant7/1 -> Divide2/2
  Constant8/1 -> Switch1/2
  IC4/1 -> Sum4/1
  Saturation3/1 -> Switch1/3, Unit Delay4/1
  Constant9/1 -> Divide3/1
  Constant10/1 -> Divide3/2
  Divide3/1 -> IC4/1
  Sum4/1 -> Saturation3/1
  Unit Delay4/1 -> Sum4/2
  Switch1/1 -> Display1/1, Mux/2

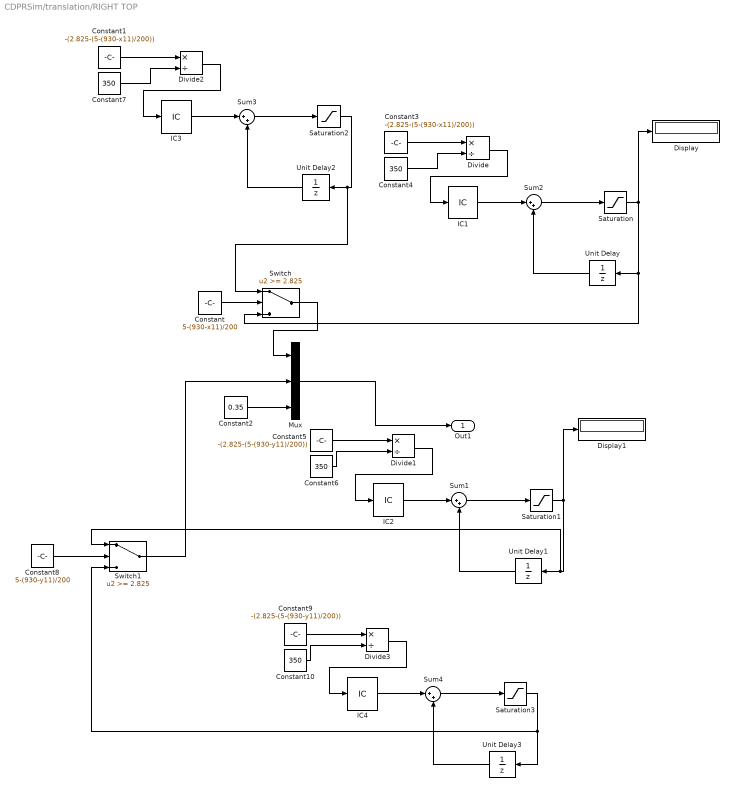
== system CDPRSim/translation/RIGHT TOP ==
  Constant : Constant  Value=5-(930-x11)/200
  Constant1 : Constant  Value=-(2.825-(5-(930-x11)/200))
  Constant{4,6..7,10} (4 alike) : Constant  Value=350
  Constant2 : Constant  Value=0.35
  Constant3 : Constant  Value=-(2.825-(5-(930-x11)/200))
  Constant5 : Constant  Value=-(2.825-(5-(930-y11)/200))
  Constant8 : Constant  Value=5-(930-y11)/200
  Constant9 : Constant  Value=-(2.825-(5-(930-y11)/200))
  Display : Display
  Display1 : Display
  Divide{,1..3} (4 alike) : Product  Inputs=*/
  IC{1..4} (4 alike) : InitialCondition  Value=2.825
  Mux : Mux  Inputs=3
  Saturation : Saturate  UpperLimit=inf  LowerLimit=5-(930-x11)/200
  Saturation1 : Saturate  UpperLimit=5-(930-y11)/200  LowerLimit=-inf
  Saturation2 : Saturate  UpperLimit=5-(930-x11)/200  LowerLimit=-inf
  Saturation3 : Saturate  UpperLimit=inf  LowerLimit=5-(930-y11)/200
  Sum{1..4} (4 alike) : Sum  Inputs=|++
  Switch : Switch  Threshold=2.825  SaturateOnIntegerOverflow=off  InputSameDT=off
  Switch1 : Switch  Threshold=2.825  SaturateOnIntegerOverflow=off  InputSameDT=off
  Unit Delay{,1..3} (4 alike) : UnitDelay  SampleTime=-1  HasFrameUpgradeWarning=on
  Out1 : Outport
  wires:
  Saturation1/1 -> Display1/1, Switch1/1, Unit Delay1/1
  Constant2/1 -> Mux/3
  Mux/1 -> Out1/1
  Saturation/1 -> Switch/3, Unit Delay/1, Display/1
  Unit Delay/1 -> Sum2/2
  IC1/1 -> Sum2/1
  Constant4/1 -> Divide/2
  Constant3/1 -> Divide/1
  Divide/1 -> IC1/1
  Sum2/1 -> Saturation/1
  Sum1/1 -> Saturation1/1
  Divide1/1 -> IC2/1
  Constant5/1 -> Divide1/1
  Constant6/1 -> Divide1/2
  IC2/1 -> Sum1/1
  Unit Delay1/1 -> Sum1/2
  Switch/1 -> Mux/1
  Constant/1 -> Switch/2
  Saturation2/1 -> Switch/1, Unit Delay2/1
  Sum3/1 -> Saturation2/1
  Constant7/1 -> Divide2/2
  IC3/1 -> Sum3/1
  Constant1/1 -> Divide2/1
  Divide2/1 -> IC3/1
  Unit Delay2/1 -> Sum3/2
  Switch1/1 -> Mux/2
  Constant8/1 -> Switch1/2
  Sum4/1 -> Saturation3/1
  Constant9/1 -> Divide3/1
  Divide3/1 -> IC4/1
  Saturation3/1 -> Unit Delay3/1, Switch1/3
  Constant10/1 -> Divide3/2
  IC4/1 -> Sum4/1
  Unit Delay3/1 -> Sum4/2

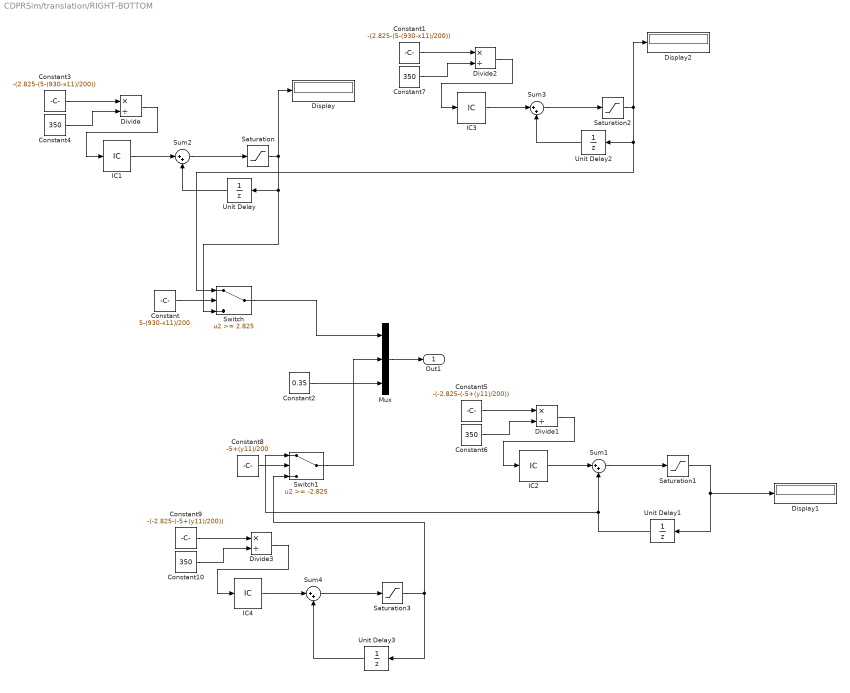
== system CDPRSim/translation/RIGHT-BOTTOM ==
  Constant : Constant  Value=5-(930-x11)/200
  Constant1 : Constant  Value=-(2.825-(5-(930-x11)/200))
  Constant{4,6..7,10} (4 alike) : Constant  Value=350
  Constant2 : Constant  Value=0.35
  Constant3 : Constant  Value=-(2.825-(5-(930-x11)/200))
  Constant5 : Constant  Value=-(-2.825-(-5+(y11)/200))
  Constant8 : Constant  Value=-5+(y11)/200
  Constant9 : Constant  Value=-(-2.825-(-5+(y11)/200))
  Display : Display
  Display1 : Display
  Display2 : Display
  Divide{,1..3} (4 alike) : Product  Inputs=*/
  IC1 : InitialCondition  Value=2.825
  IC2 : InitialCondition  Value=-2.825
  IC3 : InitialCondition  Value=2.825
  IC4 : InitialCondition  Value=-2.825
  Mux : Mux  Inputs=3
  Saturation : Saturate  UpperLimit=inf  LowerLimit=5-(930-x11)/200
  Saturation1 : Saturate  UpperLimit=-5+(y11)/200  LowerLimit=-inf
  Saturation2 : Saturate  UpperLimit=5-(930-x11)/200  LowerLimit=-inf
  Saturation3 : Saturate  UpperLimit=inf  LowerLimit=-5+(y11)/200
  Sum{1..4} (4 alike) : Sum  Inputs=|++
  Switch : Switch  Threshold=2.825  SaturateOnIntegerOverflow=off  InputSameDT=off
  Switch1 : Switch  Threshold=-2.825  SaturateOnIntegerOverflow=off  InputSameDT=off
  Unit Delay{,1..3} (4 alike) : UnitDelay  SampleTime=-1  HasFrameUpgradeWarning=on
  Out1 : Outport
  wires:
  Constant2/1 -> Mux/3
  Mux/1 -> Out1/1
  Unit Delay1/1 -> Switch1/1, Sum1/2
  IC2/1 -> Sum1/1
  Constant6/1 -> Divide1/2
  Constant5/1 -> Divide1/1
  Divide1/1 -> IC2/1
  Sum1/1 -> Saturation1/1
  Saturation1/1 -> Display1/1, Unit Delay1/1
  Sum2/1 -> Saturation/1
  Constant4/1 -> Divide/2
  IC1/1 -> Sum2/1
  Constant3/1 -> Divide/1
  Divide/1 -> IC1/1
  Saturation/1 -> Switch/3, Unit Delay/1, Display/1
  Unit Delay/1 -> Sum2/2
  Switch/1 -> Mux/1
  Constant/1 -> Switch/2
  Constant7/1 -> Divide2/2
  IC3/1 -> Sum3/1
  Sum3/1 -> Saturation2/1
  Constant1/1 -> Divide2/1
  Divide2/1 -> IC3/1
  Saturation2/1 -> Switch/1, Unit Delay2/1, Display2/1
  Unit Delay2/1 -> Sum3/2
  Switch1/1 -> Mux/2
  Constant8/1 -> Switch1/2
  Saturation3/1 -> Unit Delay3/1, Switch1/3
  Constant10/1 -> Divide3/2
  Unit Delay3/1 -> Sum4/2
  IC4/1 -> Sum4/1
  Sum4/1 -> Saturation3/1
  Divide3/1 -> IC4/1
  Constant9/1 -> Divide3/1

== system CDPRSim/Speed Module/Left bottom hız /Fark  ==
  In1 : Inport
  Display1 : Display
  Relational Operator : RelationalOperator  Operator===  OutDataTypeStr=boolean  RndMeth=Simplest  InputSameDT=off
  Sum2 : Sum  Inputs=|+-
  Triggered Subsystem1 : Subsystem  TreatAsAtomicUnit=on
  Unit Delay1 : UnitDelay  SampleTime=-1  HasFrameUpgradeWarning=on
  Out1 : Outport  VectorParamsAs1DForOutWhenUnconnected=off
  wires:
  Unit Delay1/1 -> Triggered Subsystem1/1(In1), Relational Operator/2
  Sum2/1 -> Out1/1, Display1/1
  In1/1 -> Relational Operator/1, Sum2/1, Unit Delay1/1
  Triggered Subsystem1/1(Out1) -> Sum2/2
  Relational Operator/1 -> Triggered Subsystem1/Trigger

== system CDPRSim/Speed Module/Left bottom hız /constant ==
  In1 : Inport
  Constant : Constant  Value=x11
  Constant1 : Constant  Value=y11
  Display5 : Display
  Product : Product
  Sum : Sum  Inputs=|+-
  Out1 : Outport  VectorParamsAs1DForOutWhenUnconnected=off
  wires:
  Sum/1 -> Out1/1, Display5/1
  Constant1/1 -> Sum/1
  In1/1 -> Product/1
  Constant/1 -> Product/2
  Product/1 -> Sum/2

== system CDPRSim/Speed Module/Left bottom hız /slope  ==
  In1 : Inport
  In2 : Inport  Port=2
  Divide1 : Product  Inputs=*/
  Out1 : Outport  VectorParamsAs1DForOutWhenUnconnected=off
  wires:
  Divide1/1 -> Out1/1
  In2/1 -> Divide1/2
  In1/1 -> Divide1/1

== system CDPRSim/Speed Module/Left bottom hız /x2-x1 ==
  Constant : Constant
  Display8 : Display
  Gain : Gain  Gain=x11
  Relational Operator4 : RelationalOperator  Operator===  OutDataTypeStr=boolean  RndMeth=Simplest  InputSameDT=off
  Sum5 : Sum  Inputs=|+-
  Triggered Subsystem4 : Subsystem  TreatAsAtomicUnit=on
  Unit Delay5 : UnitDelay  SampleTime=-1  HasFrameUpgradeWarning=on
  Out6 : Outport  VectorParamsAs1DForOutWhenUnconnected=off
  Out1 : Outport  Port=2  VectorParamsAs1DForOutWhenUnconnected=off
  wires:
  Gain/1 -> Sum5/1, Unit Delay5/1, Out6/1, Relational Operator4/1
  Constant/1 -> Gain/1
  Sum5/1 -> Out1/1, Display8/1
  Unit Delay5/1 -> Relational Operator4/2, Triggered Subsystem4/1(In1)
  Triggered Subsystem4/1(Out1) -> Sum5/2
  Relational Operator4/1 -> Triggered Subsystem4/Trigger

== system CDPRSim/Speed Module/Left bottom hız /y value ==
  "slope " : Inport
  "constant " : Inport  Port=2
  Display : Display
  Display1 : Display
  Display2 : Display
  Eski X : Subsystem
  Product1 : Product
  Subsystem1 : Subsystem
  Sum1 : Sum  Inputs=|++
  Out1 : Outport  VectorParamsAs1DForOutWhenUnconnected=off
  wires:
  Sum1/1 -> Out1/1
  Product1/1 -> Sum1/2
  "slope "/1 -> Product1/1
  ? -> Display1/1
  "constant "/1 -> Sum1/1
  Eski X/1(Out1) -> Display2/1, Subsystem1/1(In2), Display/1

== system CDPRSim/Speed Module/Left bottom hız /y2-y1 ==
  Constant1 : Constant
  Display1 : Display
  Gain1 : Gain  Gain=y11
  Relational Operator1 : RelationalOperator  Operator===  OutDataTypeStr=boolean  RndMeth=Simplest  InputSameDT=off
  Sum1 : Sum  Inputs=|+-
  Triggered Subsystem1 : Subsystem  TreatAsAtomicUnit=on
  Unit Delay1 : UnitDelay  SampleTime=-1  HasFrameUpgradeWarning=on
  Out1 : Outport  VectorParamsAs1DForOutWhenUnconnected=off
  Out2 : Outport  Port=2  VectorParamsAs1DForOutWhenUnconnected=off
  wires:
  Sum1/1 -> Out2/1, Display1/1
  Gain1/1 -> Out1/1, Relational Operator1/1, Unit Delay1/1, Sum1/1
  Constant1/1 -> Gain1/1
  Unit Delay1/1 -> Triggered Subsystem1/1(In1), Relational Operator1/2
  Relational Operator1/1 -> Triggered Subsystem1/Trigger
  Triggered Subsystem1/1(Out1) -> Sum1/2

== system CDPRSim/Speed Module/Left bottom hız /yeni uzunluklar  ==
  In1 : Inport
  Display1 : Display
  Display2 : Display
  Display5 : Display
  Eski X : Subsystem
  Sqrt2 : Sqrt
  Square : Math  Operator=square  SignedPower=on
  Square1 : Math  Operator=square  SignedPower=on
  Subsystem2 : Subsystem
  Sum1 : Sum  Inputs=|++
  Out1 : Outport  VectorParamsAs1DForOutWhenUnconnected=off
  wires:
  Sum1/1 -> Sqrt2/1
  Square1/1 -> Sum1/2
  Sqrt2/1 -> Display2/1, Out1/1
  Subsystem2/1(Out1) -> Display5/1, Square/1
  In1/1 -> Display1/1, Square1/1
  Square/1 -> Sum1/1
  Eski X/1(Out1) -> Subsystem2/1(In2)

== system CDPRSim/Speed Module/Subsystem/Fark  ==
  In1 : Inport
  Display1 : Display
  Relational Operator : RelationalOperator  Operator===  OutDataTypeStr=boolean  RndMeth=Simplest  InputSameDT=off
  Sum2 : Sum  Inputs=|+-
  Triggered Subsystem1 : Subsystem  TreatAsAtomicUnit=on
  Unit Delay1 : UnitDelay  SampleTime=-1  HasFrameUpgradeWarning=on
  Out1 : Outport  VectorParamsAs1DForOutWhenUnconnected=off
  wires:
  Unit Delay1/1 -> Triggered Subsystem1/1(In1), Relational Operator/2
  Sum2/1 -> Out1/1, Display1/1
  In1/1 -> Relational Operator/1, Sum2/1, Unit Delay1/1
  Triggered Subsystem1/1(Out1) -> Sum2/2
  Relational Operator/1 -> Triggered Subsystem1/Trigger

== system CDPRSim/Speed Module/Subsystem/constant ==
  In1 : Inport
  Constant : Constant
  Constant1 : Constant  Value=y11
  Constant2 : Constant
  Constant3 : Constant
  Display5 : Display
  Gain : Gain  Gain=x11
  Gain2 : Gain  Gain=1000
  Gain3 : Gain  Gain=70
  Product : Product
  Sum : Sum  Inputs=|+-
  Sum1 : Sum  Inputs=|+--
  Out1 : Outport  VectorParamsAs1DForOutWhenUnconnected=off
  wires:
  Sum/1 -> Out1/1, Display5/1
  Constant1/1 -> Sum/1
  In1/1 -> Product/1
  Sum1/1 -> Product/2
  Product/1 -> Sum/2
  Constant3/1 -> Gain3/1
  Gain3/1 -> Sum1/3
  Constant2/1 -> Gain/1
  Constant/1 -> Gain2/1
  Gain2/1 -> Sum1/1
  Gain/1 -> Sum1/2

== system CDPRSim/Speed Module/Subsystem/slope  ==
  In1 : Inport
  In2 : Inport  Port=2
  Divide1 : Product  Inputs=*/
  Out1 : Outport  VectorParamsAs1DForOutWhenUnconnected=off
  wires:
  Divide1/1 -> Out1/1
  In2/1 -> Divide1/2
  In1/1 -> Divide1/1

== system CDPRSim/Speed Module/Subsystem/x2-x1 ==
  Constant : Constant
  Constant2 : Constant
  Constant3 : Constant
  Display8 : Display
  Gain : Gain  Gain=x11
  Gain2 : Gain  Gain=1000
  Gain3 : Gain  Gain=70
  Relational Operator4 : RelationalOperator  Operator===  OutDataTypeStr=boolean  RndMeth=Simplest  InputSameDT=off
  Sum1 : Sum  Inputs=|+--
  Sum5 : Sum  Inputs=|+-
  Triggered Subsystem4 : Subsystem  TreatAsAtomicUnit=on
  Unit Delay5 : UnitDelay  SampleTime=-1  HasFrameUpgradeWarning=on
  Out6 : Outport  VectorParamsAs1DForOutWhenUnconnected=off
  Out1 : Outport  Port=2  VectorParamsAs1DForOutWhenUnconnected=off
  wires:
  Sum1/1 -> Sum5/1, Unit Delay5/1, Out6/1, Relational Operator4/1
  Sum5/1 -> Out1/1, Display8/1
  Unit Delay5/1 -> Relational Operator4/2, Triggered Subsystem4/1(In1)
  Triggered Subsystem4/1(Out1) -> Sum5/2
  Relational Operator4/1 -> Triggered Subsystem4/Trigger
  Gain/1 -> Sum1/2
  Gain2/1 -> Sum1/1
  Constant/1 -> Gain2/1
  Gain3/1 -> Sum1/3
  Constant2/1 -> Gain/1
  Constant3/1 -> Gain3/1

== system CDPRSim/Speed Module/Subsystem/y value ==
  "slope " : Inport
  "constant " : Inport  Port=2
  Eski X : Subsystem
  Product1 : Product
  Subsystem2 : Subsystem
  Sum1 : Sum  Inputs=|++
  Out1 : Outport  VectorParamsAs1DForOutWhenUnconnected=off
  wires:
  Sum1/1 -> Out1/1
  Eski X/1(Out1) -> Subsystem2/1(In2)
  Product1/1 -> Sum1/2
  "slope "/1 -> Product1/1
  Subsystem2/1(Out1) -> Product1/2
  "constant "/1 -> Sum1/1

== system CDPRSim/Speed Module/Subsystem/y2-y1 ==
  Constant1 : Constant
  Display1 : Display
  Gain1 : Gain  Gain=y11
  Relational Operator1 : RelationalOperator  Operator===  OutDataTypeStr=boolean  RndMeth=Simplest  InputSameDT=off
  Sum1 : Sum  Inputs=|+-
  Triggered Subsystem1 : Subsystem  TreatAsAtomicUnit=on
  Unit Delay1 : UnitDelay  SampleTime=-1  HasFrameUpgradeWarning=on
  Out1 : Outport  VectorParamsAs1DForOutWhenUnconnected=off
  Out2 : Outport  Port=2  VectorParamsAs1DForOutWhenUnconnected=off
  wires:
  Sum1/1 -> Out2/1, Display1/1
  Gain1/1 -> Out1/1, Relational Operator1/1, Unit Delay1/1, Sum1/1
  Constant1/1 -> Gain1/1
  Unit Delay1/1 -> Triggered Subsystem1/1(In1), Relational Operator1/2
  Relational Operator1/1 -> Triggered Subsystem1/Trigger
  Triggered Subsystem1/1(Out1) -> Sum1/2

== system CDPRSim/Speed Module/Subsystem/yeni uzunluklar  ==
  In1 : Inport
  Display1 : Display
  Display2 : Display
  Display5 : Display
  Eski X : Subsystem
  Sqrt2 : Sqrt
  Square : Math  Operator=square  SignedPower=on
  Square1 : Math  Operator=square  SignedPower=on
  Subsystem2 : Subsystem
  Sum1 : Sum  Inputs=|++
  Out1 : Outport  VectorParamsAs1DForOutWhenUnconnected=off
  wires:
  Sum1/1 -> Sqrt2/1
  Square1/1 -> Sum1/2
  Sqrt2/1 -> Display2/1, Out1/1
  Subsystem2/1(Out1) -> Display5/1, Square/1
  In1/1 -> Display1/1, Square1/1
  Square/1 -> Sum1/1
  Eski X/1(Out1) -> Subsystem2/1(In2)

== system CDPRSim/Speed Module/Left bottom hız /Fark /Triggered Subsystem1 ==
  In1 : Inport
  Trigger : TriggerPort  TriggerType=falling  VariantControl=Variant
  Out1 : Outport  VectorParamsAs1DForOutWhenUnconnected=off
  wires:
  In1/1 -> Out1/1

== system CDPRSim/Speed Module/Left bottom hız /x2-x1/Triggered Subsystem4 ==
  In1 : Inport
  Trigger : TriggerPort  TriggerType=falling  VariantControl=Variant
  Out1 : Outport  VectorParamsAs1DForOutWhenUnconnected=off
  wires:
  In1/1 -> Out1/1

== system CDPRSim/Speed Module/Left bottom hız /y value/Eski X ==
  Constant2 : Constant  Value=x11
  Relational Operator4 : RelationalOperator  Operator===  OutDataTypeStr=boolean  RndMeth=Simplest  InputSameDT=off
  Triggered Subsystem4 : Subsystem  TreatAsAtomicUnit=on
  Unit Delay5 : UnitDelay  SampleTime=-1  HasFrameUpgradeWarning=on
  Out1 : Outport  VectorParamsAs1DForOutWhenUnconnected=off
  wires:
  Relational Operator4/1 -> Triggered Subsystem4/Trigger
  Unit Delay5/1 -> Relational Operator4/2, Triggered Subsystem4/1(In1)
  Constant2/1 -> Unit Delay5/1, Relational Operator4/1
  Triggered Subsystem4/1(Out1) -> Out1/1

== system CDPRSim/Speed Module/Left bottom hız /y value/Subsystem1 ==
  In2 : Inport
  Abs : Abs  SaturateOnIntegerOverflow=off
  Abs1 : Abs  SaturateOnIntegerOverflow=off
  Constant : Constant  Value=x11
  Constant1 : Constant  Value=10000
  Constant2 : Constant  Value=10000
  Constant3 : Constant  Value=0
  Display : Display
  Display1 : Display
  Divide : Product  Inputs=*/
  Divide1 : Product  Inputs=*/
  Edit : EditField  LabelPosition=Hide  ShowInitialText=on  Alignment=Center
  Edit1 : EditField  LabelPosition=Hide  ShowInitialText=on  Alignment=Center
  Switch4 : Switch  Threshold=x11  SaturateOnIntegerOverflow=off  InputSameDT=off
  x2-x1 : Subsystem
  x2-x2 : Subsystem
  wires:
  In2/1 -> Switch4/2, Display/1
  x2-x1/1(Out2) -> Abs/1
  Abs/1 -> Divide/1
  Constant1/1 -> Divide/2
  Abs1/1 -> Divide1/1
  x2-x2/1(Out2) -> Abs1/1
  Constant2/1 -> Divide1/2
  Divide/1 -> ?
  Constant/1 -> Display1/1

== system CDPRSim/Speed Module/Left bottom hız /y2-y1/Triggered Subsystem1 ==
  In1 : Inport
  Trigger : TriggerPort  TriggerType=falling  VariantControl=Variant
  Out1 : Outport  VectorParamsAs1DForOutWhenUnconnected=off
  wires:
  In1/1 -> Out1/1

== system CDPRSim/Speed Module/Left bottom hız /yeni uzunluklar /Eski X ==
  Constant2 : Constant  Value=x11
  Relational Operator4 : RelationalOperator  Operator===  OutDataTypeStr=boolean  RndMeth=Simplest  InputSameDT=off
  Triggered Subsystem4 : Subsystem  TreatAsAtomicUnit=on
  Unit Delay5 : UnitDelay  SampleTime=-1  HasFrameUpgradeWarning=on
  Out1 : Outport  VectorParamsAs1DForOutWhenUnconnected=off
  wires:
  Relational Operator4/1 -> Triggered Subsystem4/Trigger
  Unit Delay5/1 -> Relational Operator4/2, Triggered Subsystem4/1(In1)
  Constant2/1 -> Unit Delay5/1, Relational Operator4/1
  Triggered Subsystem4/1(Out1) -> Out1/1

== system CDPRSim/Speed Module/Left bottom hız /yeni uzunluklar /Subsystem2 ==
  In2 : Inport
  Abs : Abs  SaturateOnIntegerOverflow=off
  Abs1 : Abs  SaturateOnIntegerOverflow=off
  Add : Sum
  Add1 : Sum
  Add2 : Sum
  Add3 : Sum  Inputs=+-
  Constant1 : Constant  Value=10000
  Constant2 : Constant  Value=10000
  Delay : Delay  DelayLength=1  InitialCondition=0
  Delay1 : Delay  DelayLength=1  InitialCondition=0
  Display4 : Display
  Divide : Product  Inputs=*/
  Divide1 : Product  Inputs=*/
  Saturation : Saturate  UpperLimit=x11  LowerLimit=0
  Scope1 : Scope
  Scope2 : Scope
  Switch4 : Switch  Threshold=x11  SaturateOnIntegerOverflow=off  InputSameDT=off
  x2-x1 : Subsystem
  x2-x2 : Subsystem
  Out1 : Outport  VectorParamsAs1DForOutWhenUnconnected=off
  wires:
  Switch4/1 -> Display4/1, Out1/1, Scope2/1
  Divide1/1 -> Add/1
  In2/1 -> Add3/1, Add1/1, Switch4/2
  Delay/1 -> Add/2
  Add/1 -> Delay/1, Add1/2, Scope1/1
  Delay1/1 -> Add2/2
  Divide/1 -> Add2/1
  Add2/1 -> Add3/2, Delay1/1
  Add1/1 -> Saturation/1
  Saturation/1 -> Switch4/3
  Add3/1 -> Switch4/1
  Abs/1 -> Divide/1
  x2-x1/1(Out2) -> Abs/1
  Constant1/1 -> Divide/2
  Abs1/1 -> Divide1/1
  x2-x2/1(Out2) -> Abs1/1
  Constant2/1 -> Divide1/2

== system CDPRSim/Speed Module/Subsystem/Fark /Triggered Subsystem1 ==
  In1 : Inport
  Trigger : TriggerPort  TriggerType=falling  VariantControl=Variant
  Out1 : Outport  VectorParamsAs1DForOutWhenUnconnected=off
  wires:
  In1/1 -> Out1/1

== system CDPRSim/Speed Module/Subsystem/x2-x1/Triggered Subsystem4 ==
  In1 : Inport
  Trigger : TriggerPort  TriggerType=falling  VariantControl=Variant
  Out1 : Outport  VectorParamsAs1DForOutWhenUnconnected=off
  wires:
  In1/1 -> Out1/1

== system CDPRSim/Speed Module/Subsystem/y value/Eski X ==
  Constant : Constant
  Constant2 : Constant
  Constant3 : Constant
  Gain : Gain  Gain=x11
  Gain2 : Gain  Gain=1000
  Gain3 : Gain  Gain=70
  Relational Operator4 : RelationalOperator  Operator===  OutDataTypeStr=boolean  RndMeth=Simplest  InputSameDT=off
  Sum1 : Sum  Inputs=|+--
  Triggered Subsystem4 : Subsystem  TreatAsAtomicUnit=on
  Unit Delay5 : UnitDelay  SampleTime=-1  HasFrameUpgradeWarning=on
  Out1 : Outport  VectorParamsAs1DForOutWhenUnconnected=off
  wires:
  Relational Operator4/1 -> Triggered Subsystem4/Trigger
  Unit Delay5/1 -> Relational Operator4/2, Triggered Subsystem4/1(In1)
  Sum1/1 -> Unit Delay5/1, Relational Operator4/1
  Triggered Subsystem4/1(Out1) -> Out1/1
  Constant3/1 -> Gain3/1
  Gain3/1 -> Sum1/3
  Constant2/1 -> Gain/1
  Constant/1 -> Gain2/1
  Gain2/1 -> Sum1/1
  Gain/1 -> Sum1/2

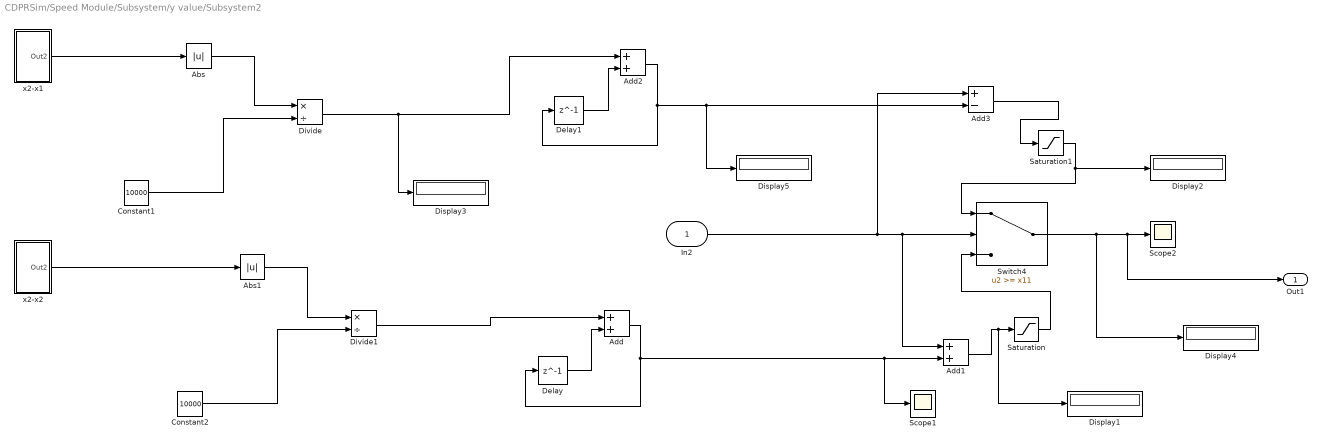
== system CDPRSim/Speed Module/Subsystem/y value/Subsystem2 ==
  In2 : Inport
  Abs : Abs  SaturateOnIntegerOverflow=off
  Abs1 : Abs  SaturateOnIntegerOverflow=off
  Add : Sum
  Add1 : Sum
  Add2 : Sum
  Add3 : Sum  Inputs=+-
  Constant1 : Constant  Value=10000
  Constant2 : Constant  Value=10000
  Delay : Delay  DelayLength=1  InitialCondition=0
  Delay1 : Delay  DelayLength=1  InitialCondition=0
  Display{1..5} (5 alike) : Display
  Divide : Product  Inputs=*/
  Divide1 : Product  Inputs=*/
  Saturation : Saturate  UpperLimit=x11  LowerLimit=0
  Saturation1 : Saturate  UpperLimit=1000  LowerLimit=x11
  Scope1 : Scope
  Scope2 : Scope
  Switch4 : Switch  Threshold=x11  SaturateOnIntegerOverflow=off  InputSameDT=off
  x2-x1 : Subsystem
  x2-x2 : Subsystem
  Out1 : Outport  VectorParamsAs1DForOutWhenUnconnected=off
  wires:
  Switch4/1 -> Display4/1, Out1/1, Scope2/1
  Divide1/1 -> Add/1
  In2/1 -> Add3/1, Add1/1, Switch4/2
  Delay/1 -> Add/2
  Add/1 -> Delay/1, Scope1/1, Add1/2
  Delay1/1 -> Add2/2
  Add3/1 -> Saturation1/1
  Add2/1 -> Delay1/1, Display5/1, Add3/2
  Add1/1 -> Display1/1, Saturation/1
  Saturation/1 -> Switch4/3
  Saturation1/1 -> Display2/1, Switch4/1
  x2-x1/1(Out2) -> Abs/1
  Divide/1 -> Display3/1, Add2/1
  Abs/1 -> Divide/1
  Constant1/1 -> Divide/2
  Abs1/1 -> Divide1/1
  x2-x2/1(Out2) -> Abs1/1
  Constant2/1 -> Divide1/2

== system CDPRSim/Speed Module/Subsystem/y2-y1/Triggered Subsystem1 ==
  In1 : Inport
  Trigger : TriggerPort  TriggerType=falling  VariantControl=Variant
  Out1 : Outport  VectorParamsAs1DForOutWhenUnconnected=off
  wires:
  In1/1 -> Out1/1

== system CDPRSim/Speed Module/Subsystem/yeni uzunluklar /Eski X ==
  Constant : Constant
  Constant2 : Constant
  Constant3 : Constant
  Gain : Gain  Gain=x11
  Gain2 : Gain  Gain=1000
  Gain3 : Gain  Gain=70
  Relational Operator4 : RelationalOperator  Operator===  OutDataTypeStr=boolean  RndMeth=Simplest  InputSameDT=off
  Sum1 : Sum  Inputs=|+--
  Triggered Subsystem4 : Subsystem  TreatAsAtomicUnit=on
  Unit Delay5 : UnitDelay  SampleTime=-1  HasFrameUpgradeWarning=on
  Out1 : Outport  VectorParamsAs1DForOutWhenUnconnected=off
  wires:
  Relational Operator4/1 -> Triggered Subsystem4/Trigger
  Unit Delay5/1 -> Relational Operator4/2, Triggered Subsystem4/1(In1)
  Sum1/1 -> Unit Delay5/1, Relational Operator4/1
  Triggered Subsystem4/1(Out1) -> Out1/1
  Constant3/1 -> Gain3/1
  Gain3/1 -> Sum1/3
  Constant2/1 -> Gain/1
  Constant/1 -> Gain2/1
  Gain2/1 -> Sum1/1
  Gain/1 -> Sum1/2
